simulink model "lorenzwaterwheel"  (R2020a)
settings: Solver=VariableStepAuto  StartTime=0.0  StopTime=100  FixedStep=0.000001  RelTol=1e-3
settings Model: Creator=chinm  LastModifiedBy=chinm

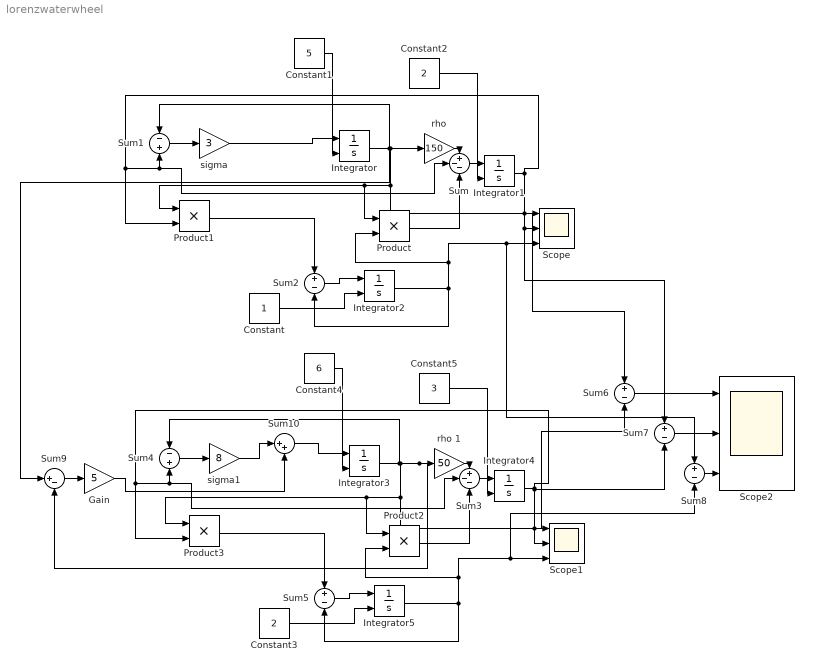
== system lorenzwaterwheel ==
  Constant : Constant
  Constant1 : Constant  Value=5
  Constant2 : Constant  Value=2
  Constant3 : Constant  Value=2
  Constant4 : Constant  Value=6
  Constant5 : Constant  Value=3
  Gain : Gain  Gain=5
  Integrator{,1..5} (6 alike) : Integrator  InitialConditionSource=external
  Product{,1..3} (4 alike) : Product
  Scope : Scope  NumInputPorts=3
  Scope1 : Scope  NumInputPorts=3
  Scope2 : Scope  NumInputPorts=3
  Sum : Sum  Inputs=+--
  Sum1 : Sum  Inputs=-+
  Sum10 : Sum  Inputs=|++
  Sum{2,5..8} (5 alike) : Sum  Inputs=+-
  Sum3 : Sum  Inputs=+--
  Sum4 : Sum  Inputs=-+
  Sum9 : Sum  Inputs=|+-
  "rho " : Gain  Gain=150
  rho 1 : Gain  Gain=50
  sigma : Gain  Gain=3
  sigma1 : Gain  Gain=8
  wires:
  Integrator/1 -> Sum9/1, Product1/1, Product/1, Sum6/1, Scope/1, "rho "/1, Sum1/1
  "rho "/1 -> Sum/1
  Sum/1 -> Integrator1/1
  Integrator1/1 -> Sum/2, Sum1/2, Product1/2, Sum7/1, Scope/2
  Sum1/1 -> sigma/1
  Integrator2/1 -> Scope/3, Sum8/1, Product/2, Sum2/2
  Product/1 -> Sum/3
  Product1/1 -> Sum2/1
  Sum2/1 -> Integrator2/1
  sigma/1 -> Integrator/1
  Constant/1 -> Integrator2/2
  Constant2/1 -> Integrator1/2
  Constant1/1 -> Integrator/2
  Constant4/1 -> Integrator3/2
  Constant3/1 -> Integrator5/2
  Product3/1 -> Sum5/1
  Integrator5/1 -> Scope1/3, Sum8/2, Product2/2, Sum5/2
  sigma1/1 -> Sum10/1
  Sum3/1 -> Integrator4/1
  Sum5/1 -> Integrator5/1
  Product2/1 -> Sum3/3
  Sum4/1 -> sigma1/1
  Constant5/1 -> Integrator4/2
  rho 1/1 -> Sum3/1
  Integrator4/1 -> Sum7/2, Scope1/2, Sum3/2, Sum4/2, Product3/2
  Integrator3/1 -> Sum9/2, rho 1/1, Product2/1, Product3/1, Sum6/2, Scope1/1, Sum4/1
  Sum8/1 -> Scope2/3
  Sum7/1 -> Scope2/2
  Sum6/1 -> Scope2/1
  Sum9/1 -> Gain/1
  Sum10/1 -> Integrator3/1
  Gain/1 -> Sum10/2
